simulink model "IterativeLearningModel"  (R2023b)
settings: Solver=VariableStepAuto  StartTime=0.0  StopTime=2.002  RelTol=1e-3
values from neighbouring files (symbols this model uses):
  feedback_den = [1    -2.832900000000000    2.672854940000000    -0.839948725176000]    [bristow_paper.m]
  feedback_num = [12.33590000000000 -35.651984590000005 34.340092218032005  -11.023646014692989]    [bristow_paper.m]
  fforward_den = fforward_den{1}    [bristow_paper.m]
  fforward_num = fforward_num{1}    [bristow_paper.m]
  plant_den = [1 -5.7154 13.723534400000000 -17.734220581599999 13.016931722320001  -5.148338416112000 0.857492875392000]    [bristow_paper.m]
  plant_num = [8.331499999999999e-04 -0.002411635990000 0.001646764298800 0.001386774757085 -0.002226794738657 7.735179924151595e-04 ]    [bristow_paper.m]
libraries: simulink x1
settings Model: Creator=Koray  LastModifiedBy=Koray

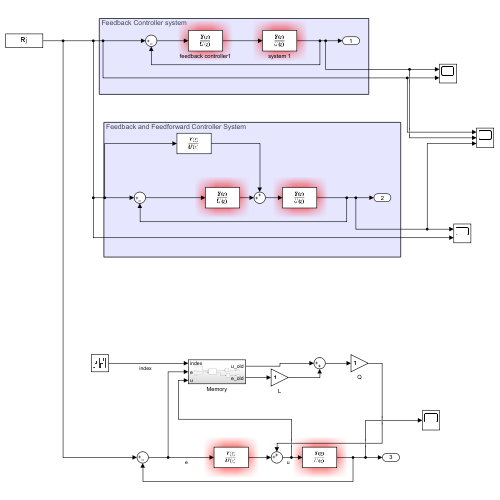
[thumbnail: Simulink's stored preview of the top-level diagram]
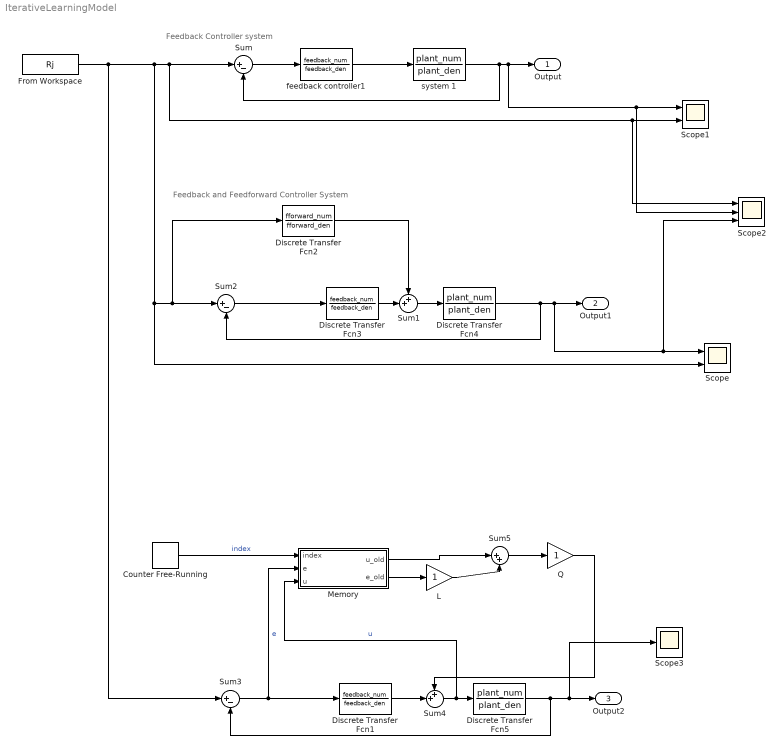
== system IterativeLearningModel ==
  note: Feedback and Feedforward Controller System
  note: Feedback Controller system
  Counter Free-Running : simulink/Sources/Counter Free-Running  NumBits=16  tsamp=0.001
  Discrete Transfer Fcn1 : DiscreteTransferFcn  Numerator=feedback_num  Denominator=feedback_den
  Discrete Transfer Fcn2 : DiscreteTransferFcn  Numerator=fforward_num  Denominator=fforward_den
  Discrete Transfer Fcn3 : DiscreteTransferFcn  Numerator=feedback_num  Denominator=feedback_den
  Discrete Transfer Fcn4 : DiscreteTransferFcn  Numerator=plant_num  Denominator=plant_den
  Discrete Transfer Fcn5 : DiscreteTransferFcn  Numerator=plant_num  Denominator=plant_den
  From Workspace : FromWorkspace  VariableName=Rj
  L : Gain
  Memory : Subsystem
  Q : Gain
  Scope : Scope  NumInputPorts=2
  Scope1 : Scope  NumInputPorts=2
  Scope2 : Scope  NumInputPorts=3
  Scope3 : Scope
  Sum : Sum  Inputs=|+-
  Sum1 : Sum  Inputs=++|
  Sum2 : Sum  Inputs=|+-
  Sum3 : Sum  Inputs=|+-
  Sum4 : Sum  Inputs=++|
  Sum5 : Sum  Inputs=|++
  feedback controller1 : DiscreteTransferFcn  Numerator=feedback_num  Denominator=feedback_den
  system 1 : DiscreteTransferFcn  Numerator=plant_num  Denominator=plant_den
  Output : Outport
  Output1 : Outport  Port=2
  Output2 : Outport  Port=3
  wires:
  Discrete Transfer Fcn3/1 -> Sum1/2
  Sum1/1 -> Discrete Transfer Fcn4/1
  Discrete Transfer Fcn2/1 -> Sum1/1
  Sum2/1 -> Discrete Transfer Fcn3/1
  Discrete Transfer Fcn4/1 -> Sum2/2, Scope2/3, Scope/1, Output1/1
  Sum/1 -> feedback controller1/1
  feedback controller1/1 -> system 1/1
  system 1/1 -> Scope2/2, Scope1/1, Output/1, Sum/2
  From Workspace/1 -> Sum3/1, Scope/2, Discrete Transfer Fcn2/1, Sum2/1, Scope2/1, Scope1/2, Sum/1
  Discrete Transfer Fcn5/1 -> Sum3/2, Scope3/1, Output2/1
  Sum3/1 -> Memory/2(e), Discrete Transfer Fcn1/1  "e"
  Discrete Transfer Fcn1/1 -> Sum4/2
  Sum4/1 -> Memory/3(u), Discrete Transfer Fcn5/1  "u"
  Counter Free-Running/1 -> Memory/1(index)  "index"
  Memory/2(e_old) -> L/1
  L/1 -> Sum5/2
  Memory/1(u_old) -> Sum5/1
  Sum5/1 -> Q/1
  Q/1 -> Sum4/1

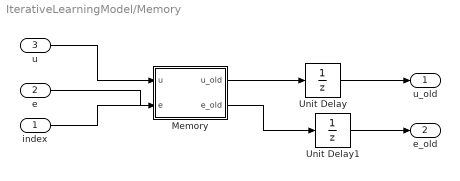
== system IterativeLearningModel/Memory ==
  index : Inport
  e : Inport  Port=2
  u : Inport  Port=3
  Memory : MATLAB Function  TreatAsAtomicUnit=on
  Unit Delay : UnitDelay  SampleTime=1.001  HasFrameUpgradeWarning=on
  Unit Delay1 : UnitDelay  SampleTime=1.001  HasFrameUpgradeWarning=on
  u_old : Outport
  e_old : Outport  Port=2
  wires:
  index/1 -> ?
  e/1 -> Memory/2(e)
  u/1 -> Memory/1(u)
  Memory/2(e_old) -> Unit Delay1/1
  Memory/1(u_old) -> Unit Delay/1
  Unit Delay1/1 -> e_old/1
  Unit Delay/1 -> u_old/1

== matlab function IterativeLearningModel/Memory/Memory ==
  data: u input; u_old output; e input; e_old output
function [u_old,e_old]  = fcn(u, e)


e_old = e;
u_old= u;
